simulink model "taller3"  (R2025b)
settings: Solver=VariableStepAuto  StartTime=0.0  StopTime=20  RelTol=1e-3
settings SolverCC: ZeroCrossAlgorithm=Adaptive
settings DebuggingCC: IgnoredZcDiagnostic=none

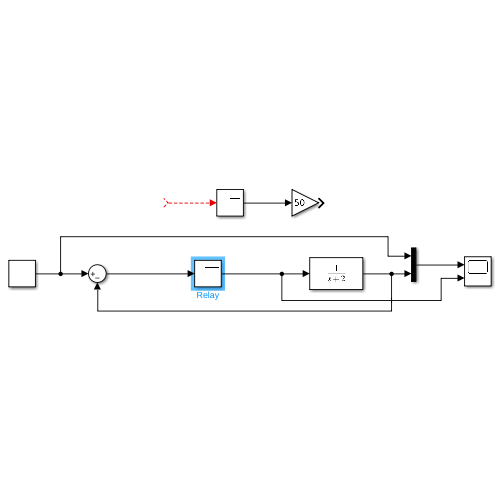
[thumbnail: Simulink's stored preview of the top-level diagram]
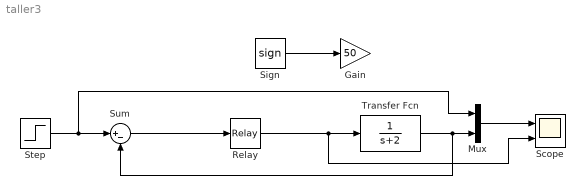
== system taller3 ==
  Gain : Gain  Gain=50
  Mux : Mux  Inputs=2
  Relay : Relay  OnSwitchValue=0.01  OffSwitchValue=-0.01  OnOutputValue=5
  Scope : Scope  NumInputPorts=2
      settings: ActiveDisplayYMinimum=-0.25125000000001579  ActiveDisplayYMaximum=2.2612500000001425
  Sign : Signum  ZeroCross=off
  Step : Step  Time=10  Before=1  After=2  SampleTime=0
  Sum : Sum  Inputs=|+-
  Transfer Fcn : TransferFcn  Denominator=[1 2]
  wires:
  Relay/1 -> Scope/2, Transfer Fcn/1
  Transfer Fcn/1 -> Sum/2, Mux/2
  Step/1 -> Mux/1, Sum/1
  Mux/1 -> Scope/1
  ? -> Sign/1
  Sign/1 -> Gain/1
  Sum/1 -> Relay/1
